simulink model "Cart_Pendulum_NonLinear_Tutor"  (R2020a)
settings: Solver=ode4  StartTime=0.0  StopTime=10.0  RelTol=1e-3
values from neighbouring files (symbols this model uses):
  A = zeros(4)    [MainFile.m]
  B = [0; 0; 1/Mc; 1/(l*Mc)]    [MainFile.m]
  C = [1, 0, 0, 0; 0, 1, 0, 0]    [MainFile.m]
  controller_enabled = 1    [MainFile.m]
  g = 9.81    [MainFile.m]
  initial_conditions = initial_conditions_b    [MainFile.m]
  K_cont = place(A, B, desiredPoles)    [MainFile.m]
  l = 0.2    [MainFile.m]
  L_obsv = place(A', C', desiredPoles)'    [MainFile.m]
  m = 0.15    [MainFile.m]
  Mc = 0.4    [MainFile.m]
  use_state_estimates = 0    [MainFile.m]
  x_bar = xb_bar    [MainFile.m]
settings Model: Creator=james  LastModifiedBy=james

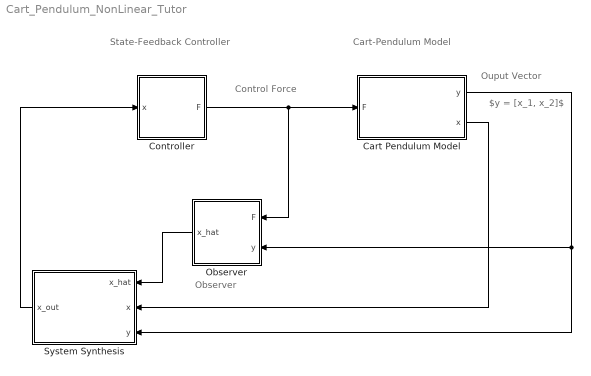
== system Cart_Pendulum_NonLinear_Tutor ==
  note: Control Force
  note: State-Feedback
      | Controller
  note: Ouput Vector
  note: Cart-Pendulum
      | Model
  note: $y = [x_1, x_2]$
  note: Observer
  Cart Pendulum Model : Subsystem
  Controller : Subsystem
  Observer : Subsystem
  System Synthesis : Subsystem
  wires:
  Controller/1(F) -> Cart Pendulum Model/1(F), Observer/1(F)
  Cart Pendulum Model/1(y) -> System Synthesis/3(y), Observer/2(y)
  Observer/1(x_hat) -> System Synthesis/1(x_hat)
  Cart Pendulum Model/2(x) -> System Synthesis/2(x)
  System Synthesis/1(x_out) -> Controller/1(x)

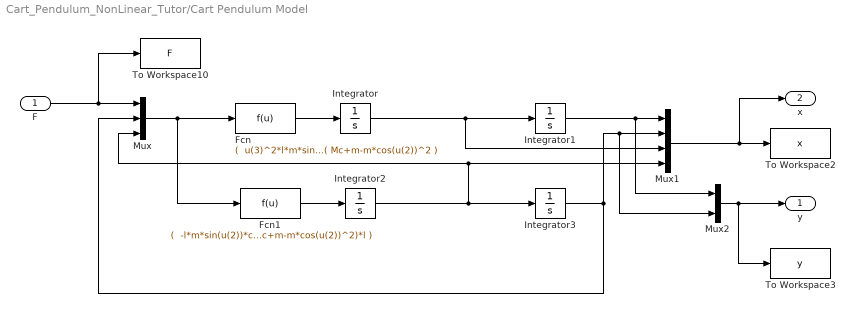
== system Cart_Pendulum_NonLinear_Tutor/Cart Pendulum Model ==
  F : Inport
  Fcn : Fcn  Expr="(  u(3)^2*l*m*sin(u(2))-g*m*sin(u(2))*cos(u(2))+u(1)) / ( Mc+m-m*cos(u(2))^2 )"
  Fcn1 : Fcn  Expr="(  -l*m*sin(u(2))*cos(u(2)) *u(3)^2   + g*(Mc+m)*sin(u(2)) - cos(u(2))*u(1)  ) / ( (Mc+m-m*cos(u(2))^2)*l )"
  Integrator : Integrator  InitialCondition=initial_conditions(3)
  Integrator1 : Integrator  InitialCondition=initial_conditions(1)
  Integrator2 : Integrator  InitialCondition=initial_conditions(4)
  Integrator3 : Integrator  InitialCondition=initial_conditions(2)
  Mux : Mux  Inputs=3
  Mux1 : Mux
  Mux2 : Mux  Inputs=2
  To Workspace10 : ToWorkspace  VariableName=F  SampleTime=-1
  To Workspace2 : ToWorkspace  VariableName=x  SampleTime=-1
  To Workspace3 : ToWorkspace  VariableName=y  SampleTime=-1
  y : Outport
  x : Outport  Port=2
  wires:
  Integrator/1 -> Mux1/3, Integrator1/1
  Integrator1/1 -> Mux2/1, Mux1/1
  Fcn1/1 -> Integrator2/1
  Mux/1 -> Fcn1/1, Fcn/1
  Integrator2/1 -> Mux1/4, Mux/3, Integrator3/1
  Mux1/1 -> x/1, To Workspace2/1
  F/1 -> To Workspace10/1, Mux/1
  Integrator3/1 -> Mux2/2, Mux1/2, Mux/2
  Fcn/1 -> Integrator/1
  Mux2/1 -> To Workspace3/1, y/1

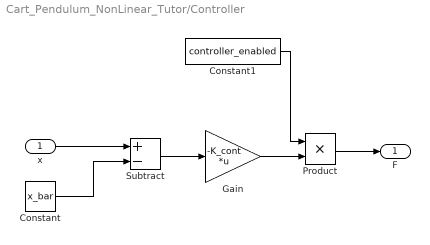
== system Cart_Pendulum_NonLinear_Tutor/Controller ==
  x : Inport
  Constant : Constant  Value=x_bar
  Constant1 : Constant  Value=controller_enabled
  Gain : Gain  Gain=-K_cont  Multiplication=Matrix(K*u)
  Product : Product
  Subtract : Sum  Inputs=+-
  F : Outport
  wires:
  Subtract/1 -> Gain/1
  x/1 -> Subtract/1
  Constant/1 -> Subtract/2
  Gain/1 -> Product/2
  Constant1/1 -> Product/1
  Product/1 -> F/1

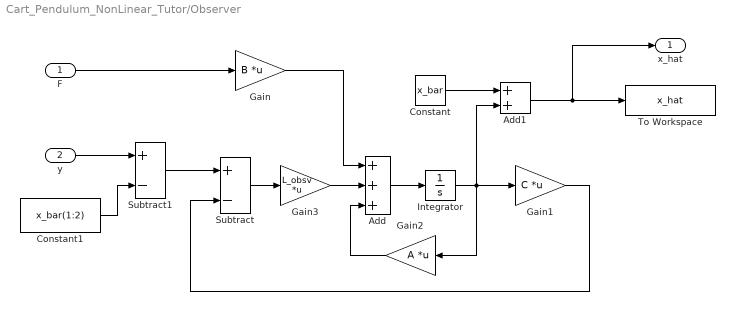
== system Cart_Pendulum_NonLinear_Tutor/Observer ==
  F : Inport
  y : Inport  Port=2
  Add : Sum  Inputs=3
  Add1 : Sum
  Constant : Constant  Value=x_bar
  Constant1 : Constant  Value=x_bar(1:2)
  Gain : Gain  Gain=B  Multiplication=Matrix(K*u)
  Gain1 : Gain  Gain=C  Multiplication=Matrix(K*u)
  Gain2 : Gain  Gain=A  Multiplication=Matrix(K*u)
  Gain3 : Gain  Gain=L_obsv  Multiplication=Matrix(K*u)
  Integrator : Integrator
  Subtract : Sum  Inputs=+-
  Subtract1 : Sum  Inputs=+-
  To Workspace : ToWorkspace  VariableName=x_hat  SampleTime=-1
  x_hat : Outport
  wires:
  F/1 -> Gain/1
  Gain/1 -> Add/1
  Gain1/1 -> Subtract/2
  Gain2/1 -> Add/3
  Add/1 -> Integrator/1
  Integrator/1 -> Add1/2, Gain2/1, Gain1/1
  Gain3/1 -> Add/2
  Subtract/1 -> Gain3/1
  Add1/1 -> To Workspace/1, x_hat/1
  Constant/1 -> Add1/1
  y/1 -> Subtract1/1
  Subtract1/1 -> Subtract/1
  Constant1/1 -> Subtract1/2

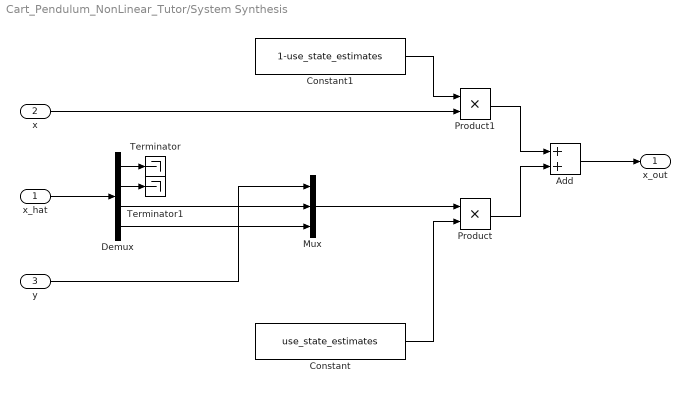
== system Cart_Pendulum_NonLinear_Tutor/System Synthesis ==
  x_hat : Inport
  x : Inport  Port=2
  y : Inport  Port=3
  Add : Sum
  Constant : Constant  Value=use_state_estimates
  Constant1 : Constant  Value=1-use_state_estimates
  Demux : Demux
  Mux : Mux  Inputs=3
  Product : Product
  Product1 : Product
  Terminator : Terminator
  Terminator1 : Terminator
  x_out : Outport
  wires:
  Demux/2 -> Terminator1/1
  Demux/1 -> Terminator/1
  x_hat/1 -> Demux/1
  y/1 -> Mux/1
  Demux/3 -> Mux/2
  Demux/4 -> Mux/3
  Constant/1 -> Product/2
  Mux/1 -> Product/1
  Constant1/1 -> Product1/1
  x/1 -> Product1/2
  Add/1 -> x_out/1
  Product1/1 -> Add/1
  Product/1 -> Add/2
